simulink model "Wheelspeed"  (R2015b)
settings: Solver=FixedStepAuto  StartTime=0.0  StopTime=100.0  RelTol=1e-3
libraries: arduinolib x12, simulink x5
settings Model: SimulationMode=external  ExtModeTrigDuration=2  Creator=Joern  LastModifiedBy=Joern
settings OptimizationCC: OptimizeModelRefInitCode=on  LifeSpan=1  MaxStackSize=64
settings HardwareCC: ProdBitPerInt=16  ProdBitPerPointer=16  ProdLargestAtomicFloat=None  ProdWordSize=8  ProdHWDeviceType=Atmel->AVR
settings RTWCC: SystemTargetFile=ert.tlc  TemplateMakefile=ert_default_tmf  Description=Embedded Coder  Toolchain=Arduino AVR v1.6.1  BuildConfiguration=Faster Runs
settings CodeAppCC: IgnoreCustomStorageClasses=off
settings ERTTargetCC: GenerateSampleERTMain=on  SupportContinuousTime=on  SupportVariableSizeSignals=on

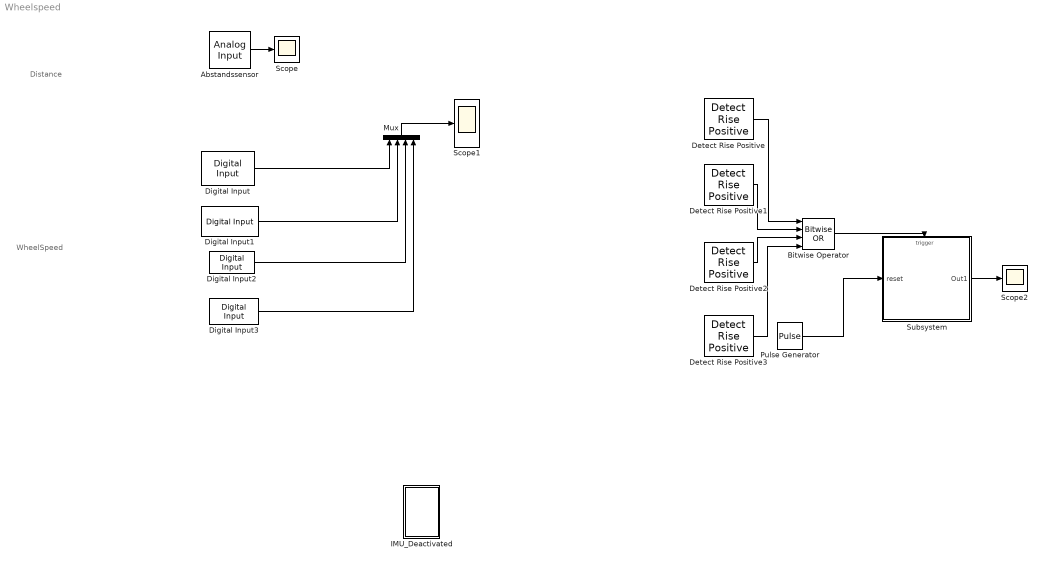
== system Wheelspeed ==
  note: WheelSpeed
  note: Distance
  Abstandssensor : arduinolib/Analog Input  pinNumber=6  sampleTime=0.1  blockPlatform=arduino
  Bitwise Operator : simulink/Logic and Bit Operations/Bitwise Operator  logicop=OR  UseBitMask=off  NumInputPorts=4  BitMask=bin2dec('11011001')  BitMaskRealWorld=Stored Integer
  Detect Rise Positive{,1..3} (4 alike) : simulink/Logic and Bit Operations/Detect Rise Positive  vinit=0  InputProcessing=Inherited  OutDataTypeStr=boolean
  Digital Input : arduinolib/Digital Input  pinNumber=18  sampleTime=0.01  blockPlatform=arduino
  Digital Input1 : arduinolib/Digital Input  pinNumber=19  sampleTime=0.01  blockPlatform=arduino
  Digital Input2 : arduinolib/Digital Input  pinNumber=2  sampleTime=0.01  blockPlatform=arduino
  Digital Input3 : arduinolib/Digital Input  pinNumber=3  sampleTime=0.01  blockPlatform=arduino
  IMU_Deactivated : Subsystem
  Mux : Mux
  Pulse Generator : DiscretePulseGenerator  PulseType=Time based  Period=1
  Scope : Scope
  Scope1 : Scope
  Scope2 : Scope
  Subsystem : Subsystem
  wires:
  Abstandssensor/1 -> Scope/1
  Mux/1 -> Scope1/1
  Digital Input/1 -> Mux/1
  Digital Input1/1 -> Mux/2
  Digital Input2/1 -> Mux/3
  Digital Input3/1 -> Mux/4
  Detect Rise Positive/1 -> Bitwise Operator/1
  Detect Rise Positive1/1 -> Bitwise Operator/2
  Detect Rise Positive2/1 -> Bitwise Operator/3
  Detect Rise Positive3/1 -> Bitwise Operator/4
  Bitwise Operator/1 -> Subsystem/Trigger
  Pulse Generator/1 -> Subsystem/1(reset)
  Subsystem/1(Out1) -> Scope2/1

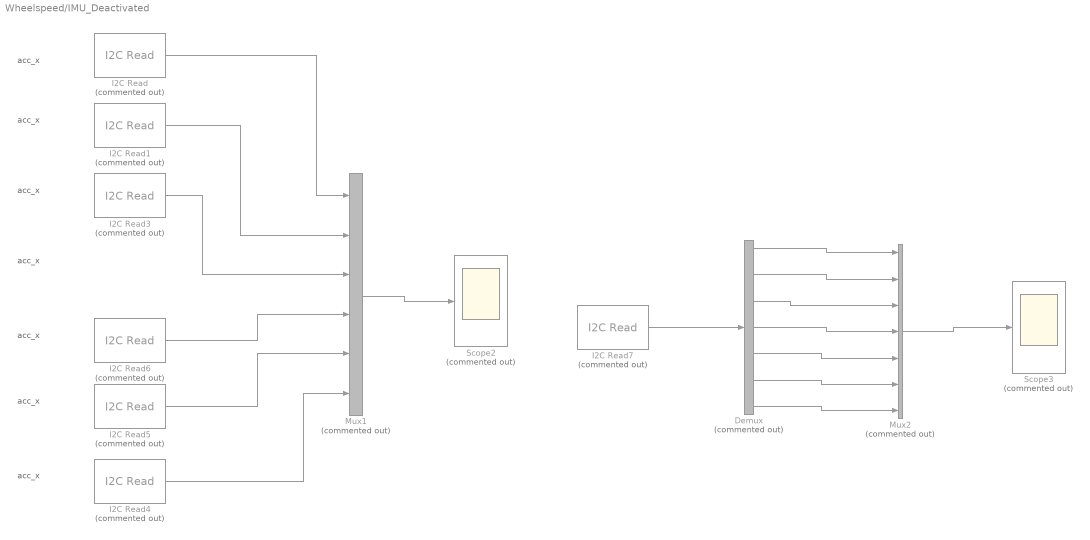
== system Wheelspeed/IMU_Deactivated ==
  note: acc_x
  note: acc_x
  note: acc_x
  note: acc_x
  note: acc_x
  note: acc_x
  note: acc_x
  Demux : Demux  Commented=on  Outputs=7
  I2C Read : arduinolib/I2C Read  Commented=on  SlaveAddress_=hex2dec( '68' )  RegisterAddressEnable=on  RegisterAddress_=hex2dec( '3B' )  Datatype=uint16  ByteOrder=Little Endian  Datalength_=1  SampleTime_=1  blockPlatform=arduino
  I2C Read1 : arduinolib/I2C Read  Commented=on  SlaveAddress_=hex2dec( '68' )  RegisterAddressEnable=on  RegisterAddress_=hex2dec( '3D' )  Datatype=uint16  ByteOrder=Little Endian  Datalength_=1  SampleTime_=1  blockPlatform=arduino
  I2C Read3 : arduinolib/I2C Read  Commented=on  SlaveAddress_=hex2dec( '68' )  RegisterAddressEnable=on  RegisterAddress_=hex2dec( '3F' )  Datatype=uint16  ByteOrder=Little Endian  Datalength_=1  SampleTime_=1  blockPlatform=arduino
  I2C Read4 : arduinolib/I2C Read  Commented=on  SlaveAddress_=hex2dec( '68' )  RegisterAddressEnable=on  RegisterAddress_=hex2dec( '47' )  Datatype=uint16  ByteOrder=Little Endian  Datalength_=1  SampleTime_=1  blockPlatform=arduino
  I2C Read5 : arduinolib/I2C Read  Commented=on  SlaveAddress_=hex2dec( '68' )  RegisterAddressEnable=on  RegisterAddress_=hex2dec( '45' )  Datatype=uint16  ByteOrder=Little Endian  Datalength_=1  SampleTime_=1  blockPlatform=arduino
  I2C Read6 : arduinolib/I2C Read  Commented=on  SlaveAddress_=hex2dec( '68' )  RegisterAddressEnable=on  RegisterAddress_=hex2dec( '43' )  Datatype=uint16  ByteOrder=Little Endian  Datalength_=1  SampleTime_=1  blockPlatform=arduino
  I2C Read7 : arduinolib/I2C Read  Commented=on  SlaveAddress_=hex2dec( '68' )  RegisterAddressEnable=off  RegisterAddress_=hex2dec( '3B' )  Datatype=uint16  ByteOrder=Little Endian  Datalength_=14  SampleTime_=0.01  blockPlatform=arduino
  Mux1 : Mux  Commented=on  Inputs=6
  Mux2 : Mux  Commented=on  Inputs=7
  Scope2 : Scope  Commented=on
  Scope3 : Scope  Commented=on
  wires:
  I2C Read6/1 -> Mux1/4
  I2C Read7/1 -> Demux/1
  Demux/3 -> Mux2/3
  I2C Read1/1 -> Mux1/2
  I2C Read/1 -> Mux1/1
  Demux/5 -> Mux2/5
  Demux/6 -> Mux2/6
  I2C Read3/1 -> Mux1/3
  Demux/1 -> Mux2/1
  I2C Read4/1 -> Mux1/6
  Mux1/1 -> Scope2/1
  Demux/2 -> Mux2/2
  Demux/4 -> Mux2/4
  I2C Read5/1 -> Mux1/5
  Mux2/1 -> Scope3/1
  Demux/7 -> Mux2/7

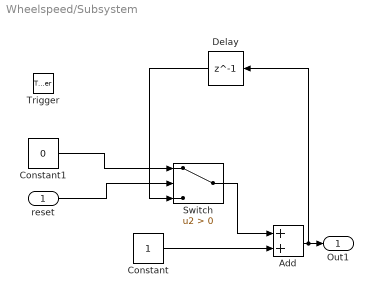
== system Wheelspeed/Subsystem ==
  reset : Inport
  Trigger : TriggerPort  PortDimensions=1
  Add : Sum  Inputs=2
  Constant : Constant
  Constant1 : Constant  Value=0
  Delay : Delay  DelayLength=1  InitialCondition=0
  Switch : Switch  Criteria=u2 > Threshold
  Out1 : Outport
  wires:
  Add/1 -> Delay/1, Out1/1
  Constant/1 -> Add/2
  reset/1 -> Switch/2
  Constant1/1 -> Switch/1
  Switch/1 -> Add/1
  Delay/1 -> Switch/3
